simulink model "simulink_youla_control101"  (R2023b)
settings: Solver=VariableStepAuto  StartTime=0.0  StopTime=endtime  RelTol=1e-3
undefined symbols (not defined in the file or in its folder): deadtime, deadtimem, Rnd, Rrd, tplot, Ts
libraries: cstblocks x4
settings Model: Creator=barsr  LastModifiedBy=barsr

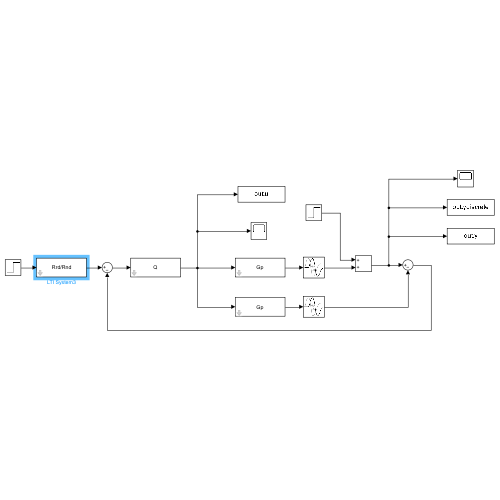
[thumbnail: Simulink's stored preview of the top-level diagram]
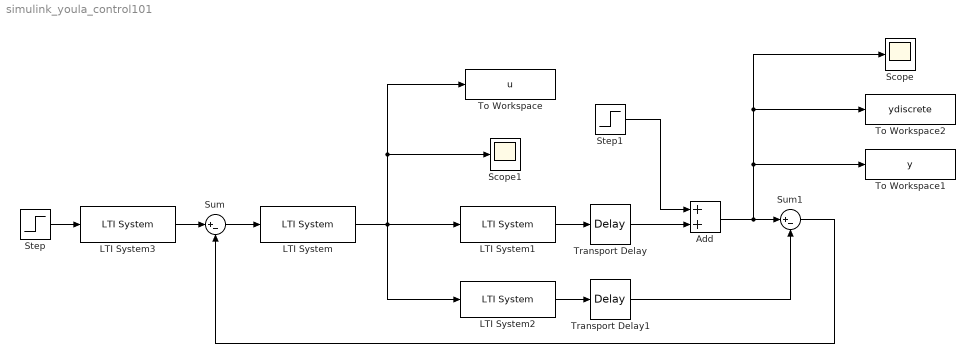
== system simulink_youla_control101 ==
  Add : Sum
  LTI System : cstblocks/LTI System  sys=Q  IC=[]  PadeOrder=0
  LTI System1 : cstblocks/LTI System  sys=Gp  IC=[]  PadeOrder=0
  LTI System2 : cstblocks/LTI System  sys=Gp  IC=[]  PadeOrder=0
  LTI System3 : cstblocks/LTI System  sys=Rrd/Rnd  IC=[]  PadeOrder=0
  Scope : Scope
  Scope1 : Scope
  Step : Step  Time=0  SampleTime=0
  Step1 : Step  Time=100  After=0.5  SampleTime=0
  Sum : Sum  Inputs=|+-
  Sum1 : Sum  Inputs=|+-
  To Workspace : ToWorkspace  VariableName=u  SaveFormat=Structure With Time  SampleTime=tplot
  To Workspace1 : ToWorkspace  VariableName=y  SaveFormat=Structure With Time  SampleTime=tplot
  To Workspace2 : ToWorkspace  VariableName=ydiscrete  SaveFormat=Structure With Time  SampleTime=Ts
  Transport Delay : TransportDelay  DelayTime=deadtime
  Transport Delay1 : TransportDelay  DelayTime=deadtimem
  wires:
  Step/1 -> LTI System3/1
  Sum/1 -> LTI System/1
  LTI System1/1 -> Transport Delay/1
  LTI System/1 -> LTI System2/1, To Workspace/1, Scope1/1, LTI System1/1
  LTI System2/1 -> Transport Delay1/1
  LTI System3/1 -> Sum/1
  Transport Delay1/1 -> Sum1/2
  Transport Delay/1 -> Add/2
  Step1/1 -> Add/1
  Add/1 -> Scope/1, To Workspace2/1, To Workspace1/1, Sum1/1
  Sum1/1 -> Sum/2
